simulink model "Sample_v_0_2"  (R2021b)
settings: Solver=VariableStepAuto  StartTime=0.0  StopTime=10.0  RelTol=1e-3
values from neighbouring files (symbols this model uses):
  KeyOff = 0    [Sample_v_0_1_Parameter.m]
  Two = 2    [Sample_v_0_1_Parameter.m]
undefined symbols (not defined in the file or in its folder): Four_bb, SystemOn
settings Model: Creator=ygkwon  LastModifiedBy=ygkwon

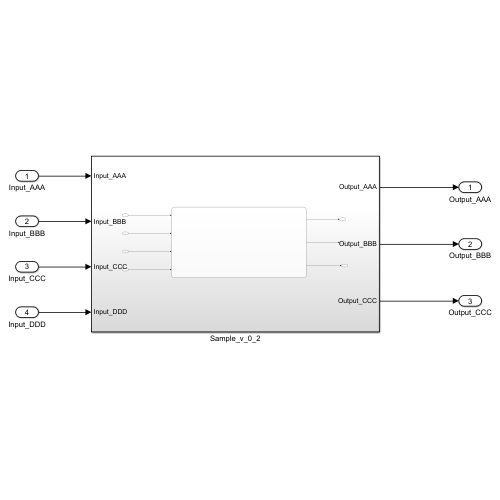
[thumbnail: Simulink's stored preview of the top-level diagram]
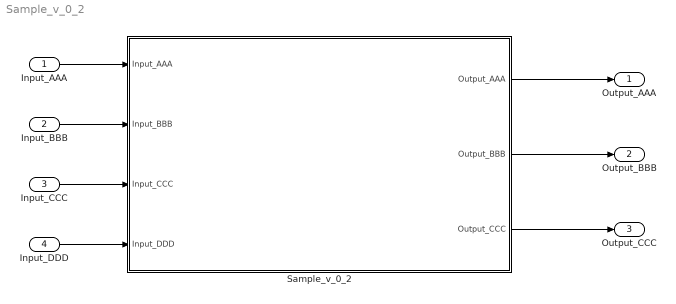
== system Sample_v_0_2 ==
  Input_AAA : Inport
  Input_BBB : Inport  Port=2
  Input_CCC : Inport  Port=3
  Input_DDD : Inport  Port=4
  Sample_v_0_2 : Subsystem
  Output_AAA : Outport
  Output_BBB : Outport  Port=2
  Output_CCC : Outport  Port=3
  wires:
  Input_AAA/1 -> Sample_v_0_2/1(Input_AAA)
  Input_BBB/1 -> Sample_v_0_2/2(Input_BBB)
  Input_CCC/1 -> Sample_v_0_2/3(Input_CCC)
  Input_DDD/1 -> Sample_v_0_2/4(Input_DDD)
  Sample_v_0_2/1(Output_AAA) -> Output_AAA/1
  Sample_v_0_2/2(Output_BBB) -> Output_BBB/1
  Sample_v_0_2/3(Output_CCC) -> Output_CCC/1

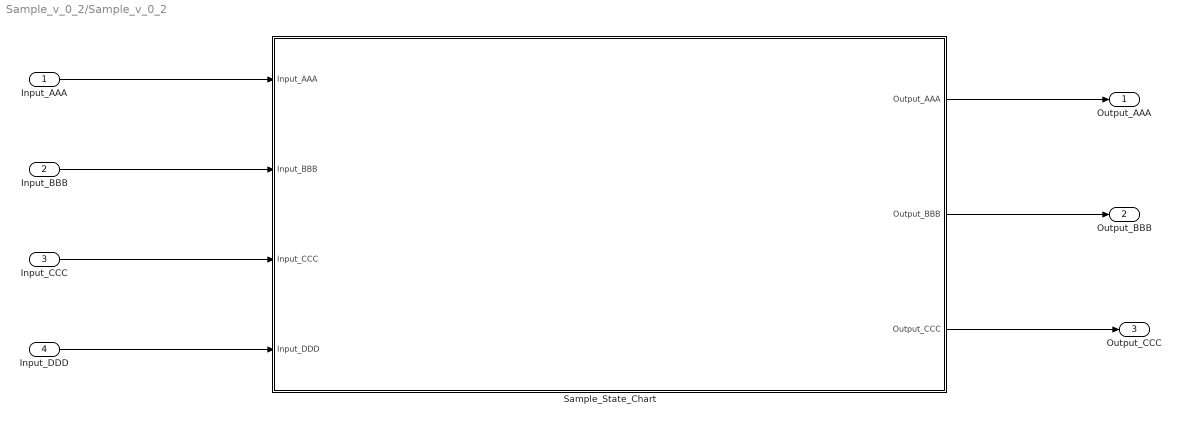
== system Sample_v_0_2/Sample_v_0_2 ==
  Input_AAA : Inport
  Input_BBB : Inport  Port=2
  Input_CCC : Inport  Port=3
  Input_DDD : Inport  Port=4
  Sample_State_Chart : Stateflow chart  TreatAsAtomicUnit=on
  Output_AAA : Outport
  Output_BBB : Outport  Port=2
  Output_CCC : Outport  Port=3
  wires:
  Input_BBB/1 -> Sample_State_Chart/2(Input_BBB)
  Input_CCC/1 -> Sample_State_Chart/3(Input_CCC)
  Input_DDD/1 -> Sample_State_Chart/4(Input_DDD)
  Sample_State_Chart/1(Output_AAA) -> Output_AAA/1
  Sample_State_Chart/2(Output_BBB) -> Output_BBB/1
  Sample_State_Chart/3(Output_CCC) -> Output_CCC/1
  Input_AAA/1 -> Sample_State_Chart/1(Input_AAA)

== stateflow chart Sample_v_0_2/Sample_State_Chart ==
  state Sample_State_Chart
    state Stop
      en:
      Output_AAA = Four_bb;
      b_Running = Off;
    state Start
      Output_AAA = Two;
      b_Running = On;
    (default) -> Stop
    Stop -> Start : [Input_AAA==SystemOn]
    Start -> Stop : [Input_AAA==Four_bb]
  state Test_for [function]
    (default) -> (junction 28)
    (junction 28) -> (junction 32) [order 2] : [Input_CCC == Four_bb]
    (junction 28) -> (junction 30) [order 1]
    (junction 32) -> (junction 33)
    (junction 33) -> (junction 30)
    (junction 30) -> (junction 37)
  (default) -> Sample_State_Chart
  data: Input_AAA input uint8; Input_BBB input uint8; Input_CCC input uint8; Input_DDD input uint8; Output_AAA output uint8; Output_BBB output uint8; Output_CCC output uint8; Four_bb parameter uint8; Two parameter uint8; SystemOn parameter uint8; KeyOff parameter uint8; b_Running local boolean; On parameter boolean; Off parameter boolean
